simulink model "washout_estimator"  (R2017b)
settings: Solver=FixedStepDiscrete  StartTime=0.0  StopTime=T  FixedStep=0.01  RelTol=1e-3
values from neighbouring files (symbols this model uses):
  Cf = 100000    [Init_for_washout_filter.m]
  Cr = 100000    [Init_for_washout_filter.m]
  L = lf+lr    (= 2.55)    [Init_for_washout_filter.m]
  lf = 0.41*2.55    (= 1.0455)    [Init_for_washout_filter.m]
  lr = 2.55-lf    (= 1.5045)    [Init_for_washout_filter.m]
  mass = 1435-80    (= 1355)    [Init_for_washout_filter.m]
  rollGrad = 5*(pi/180)    (= 0.0872664625997)    [Init_for_washout_filter.m]
  T_w = 1    [mainscript.m]
undefined symbols (not defined in the file or in its folder): DiscIntNeverNeededParam
settings Model: Creator=gandh  LastModifiedBy=gandh

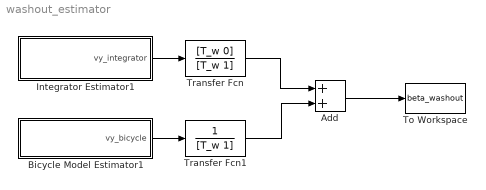
== system washout_estimator ==
  Add : Sum
  Bicycle Model Estimator1 : Subsystem
  Integrator Estimator1 : Subsystem
  To Workspace : ToWorkspace  VariableName=beta_washout  SaveFormat=Timeseries  SampleTime=-1
  Transfer Fcn : TransferFcn  Numerator=[T_w 0]  Denominator=[T_w 1]
  Transfer Fcn1 : TransferFcn  Denominator=[T_w 1]
  wires:
  Integrator Estimator1/1(vy_integrator) -> Transfer Fcn/1
  Bicycle Model Estimator1/1(vy_bicycle) -> Transfer Fcn1/1
  Add/1 -> To Workspace/1
  Transfer Fcn/1 -> Add/1
  Transfer Fcn1/1 -> Add/2

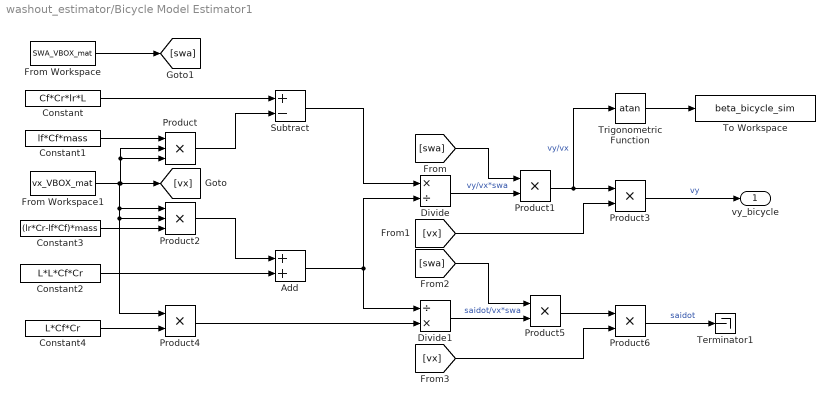
== system washout_estimator/Bicycle Model Estimator1 ==
  Add : Sum
  Constant : Constant  Value=Cf*Cr*lr*L
  Constant1 : Constant  Value=lf*Cf*mass
  Constant2 : Constant  Value=L*L*Cf*Cr
  Constant3 : Constant  Value=(lr*Cr-lf*Cf)*mass
  Constant4 : Constant  Value=L*Cf*Cr
  Divide : Product  Inputs=*/
  Divide1 : Product  Inputs=/*
  From Workspace : FromWorkspace  VariableName=SWA_VBOX_mat  SampleTime=0
  From Workspace1 : FromWorkspace  VariableName=vx_VBOX_mat  SampleTime=0
  Product : Product  Inputs=3
  Product{1,3..6} (5 alike) : Product
  Product2 : Product  Inputs=3
  Subtract : Sum  Inputs=+-
  Terminator1 : Terminator
  To Workspace : ToWorkspace  VariableName=beta_bicycle_sim  SaveFormat=Timeseries  SampleTime=-1
  Trigonometric Function : Trigonometry  Operator=atan
  vy_bicycle : Outport
  wires:
  Product4/1 -> Divide1/2
  [swa] -> Product5/1
  [vx] -> Product6/2
  Subtract/1 -> Divide/1
  Product2/1 -> Add/1
  Product5/1 -> Product6/1
  Constant3/1 -> Product2/3
  Product/1 -> Subtract/2
  Divide/1 -> Product1/2  "vy/vx*swa"
  From Workspace/1 -> [swa]
  Constant4/1 -> Product4/2
  Constant1/1 -> Product/1
  Product6/1 -> Terminator1/1  "saidot"
  From Workspace1/1 -> Product/2, Product/3, [vx], Product2/1, Product4/1, Product2/2
  [swa] -> Product1/1
  Divide1/1 -> Product5/2  "saidot/vx*swa"
  Product3/1 -> vy_bicycle/1  "vy"
  Constant/1 -> Subtract/1
  Trigonometric Function/1 -> To Workspace/1
  Add/1 -> Divide/2, Divide1/1
  Product1/1 -> Product3/1, Trigonometric Function/1  "vy/vx"
  Constant2/1 -> Add/2
  [vx] -> Product3/2

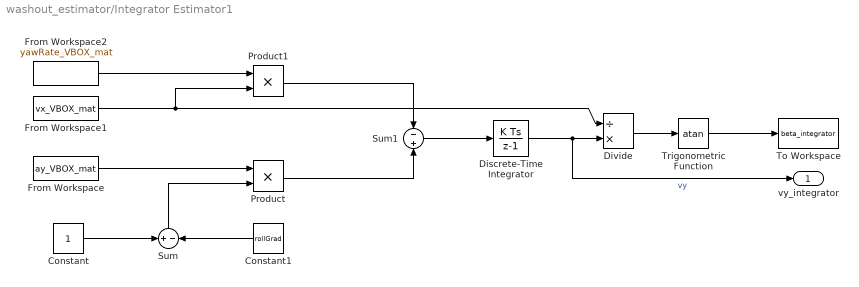
== system washout_estimator/Integrator Estimator1 ==
  Constant : Constant
  Constant1 : Constant  Value=rollGrad
  Discrete-Time Integrator : DiscreteIntegrator  InitialConditionSetting=State (most efficient)  SampleTime=-1  ICPrevOutput=DiscIntNeverNeededParam  ICPrevScaledInput=DiscIntNeverNeededParam
  Divide : Product  Inputs=/*
  From Workspace : FromWorkspace  VariableName=ay_VBOX_mat  SampleTime=0
  From Workspace1 : FromWorkspace  VariableName=vx_VBOX_mat  SampleTime=0
  From Workspace2 : FromWorkspace  VariableName=yawRate_VBOX_mat  SampleTime=0
  Product : Product
  Product1 : Product
  Sum : Sum  Inputs=+-
  Sum1 : Sum  Inputs=-+
  To Workspace : ToWorkspace  VariableName=beta_integrator  SaveFormat=Timeseries  SampleTime=-1
  Trigonometric Function : Trigonometry  Operator=atan
  vy_integrator : Outport
  wires:
  Sum/1 -> Product/2
  Sum1/1 -> Discrete-Time Integrator/1
  Divide/1 -> Trigonometric Function/1
  Product1/1 -> Sum1/1
  From Workspace2/1 -> Product1/1
  Constant1/1 -> Sum/2
  Product/1 -> Sum1/2
  Constant/1 -> Sum/1
  From Workspace1/1 -> Product1/2, Divide/1
  From Workspace/1 -> Product/1
  Trigonometric Function/1 -> To Workspace/1
  Discrete-Time Integrator/1 -> vy_integrator/1, Divide/2  "vy"
